simulink model "mconversion9"  (Simulink 6.0)
settings: Solver=FixedStepDiscrete  StartTime=0.0  StopTime=10.0  RelTol=1e-3
settings Model: Creator=awarlock  LastModifiedBy=awarlock  ExtModeAutoUpdateStatusClock=off
settings OptimizationCC: InlineParams=on
settings DebuggingCC: CheckExecutionContextPreStartOutputMsg=on  CheckExecutionContextRuntimeOutputMsg=on
settings SFSimCC: SFSimApplyToAllLibs=on  SFSimBuildMode=Incremental

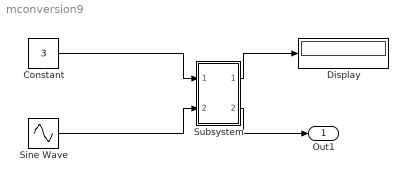
== system mconversion9 ==
  Constant : Constant  Value=3
  Display : Display
  Sine Wave : Sin  SampleTime=0.1
  Subsystem : Subsystem  TreatAsAtomicUnit=on  PropExecContextAcrossSSBoundary=on
  Out1 : Outport
  wires:
  Constant/1 -> Subsystem/1(In1)
  Sine Wave/1 -> Subsystem/2(In2)
  Subsystem/2(Out2) -> Out1/1
  Subsystem/1(Out1) -> Display/1

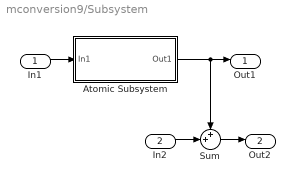
== system mconversion9/Subsystem ==
  In1 : Inport  LatchInput=off
  In2 : Inport  Port=2  LatchInput=off
  Atomic Subsystem : Subsystem  TreatAsAtomicUnit=on  PropExecContextAcrossSSBoundary=on
  Sum : Sum  Inputs=++|
  Out1 : Outport
  Out2 : Outport  Port=2
  wires:
  Atomic Subsystem/1(Out1) -> Sum/1, Out1/1
  In1/1 -> Atomic Subsystem/1(In1)
  In2/1 -> Sum/2
  Sum/1 -> Out2/1

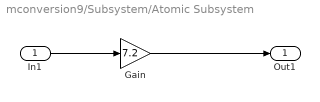
== system mconversion9/Subsystem/Atomic Subsystem ==
  In1 : Inport  LatchInput=off
  Gain : Gain  Gain=7.2
  Out1 : Outport
  wires:
  In1/1 -> Gain/1
  Gain/1 -> Out1/1
